simulink model "FSAC2021_V1_Running"  (R2014a)
settings: Solver=FixedStepDiscrete  StartTime=0.0  StopTime=inf  FixedStep=0.0005  RelTol=1e-3
model workspace (MAT data in the model file):
  MCOS : class17 (value not decoded)
  MCOS : class17 (value not decoded)
  MCOS : class17 (value not decoded)
  MCOS : class17 (value not decoded)
  MCOS : class17 (value not decoded)
  MCOS : class17 (value not decoded)
  MCOS : class17 (value not decoded)
  MCOS : class17 (value not decoded)
  MCOS : class17 (value not decoded)
  MCOS : class17 (value not decoded)
  MCOS : class17 (value not decoded)
  MCOS : class17 (value not decoded)
  MCOS : class17 (value not decoded)
  MCOS : class17 (value not decoded)
  MCOS : class17 (value not decoded)
  MCOS : class17 (value not decoded)
  MCOS : class17 (value not decoded)
  MCOS : class17 (value not decoded)
  MCOS : class17 (value not decoded)
  BUZZER_START = 1
  MCOS : class17 (value not decoded)
  MCOS : class17 (value not decoded)
  MCOS : class17 (value not decoded)
  MCOS : class17 (value not decoded)
  MCOS : class17 (value not decoded)
  MCOS : class17 (value not decoded)
  MCOS : class17 (value not decoded)
  MCOS : class17 (value not decoded)
  MCOS : class17 (value not decoded)
  MCOS : class17 (value not decoded)
  MCOS : class17 (value not decoded)
  MCOS : class17 (value not decoded)
  MCOS : class17 (value not decoded)
  MCOS : class17 (value not decoded)
  MCOS : class17 (value not decoded)
  MCOS : class17 (value not decoded)
  MCOS : class17 (value not decoded)
  MCOS : class17 (value not decoded)
  MCOS : class17 (value not decoded)
  MCOS : class17 (value not decoded)
  MCOS : class17 (value not decoded)
  MCOS : class17 (value not decoded)
  MCOS : class17 (value not decoded)
  MCOS : class17 (value not decoded)
  MCOS : class17 (value not decoded)
  MCOS : class17 (value not decoded)
  MCOS : class17 (value not decoded)
  MCOS : class17 (value not decoded)
  MCOS : class17 (value not decoded)
  MCOS : class17 (value not decoded)
  MCOS : class17 (value not decoded)
  MCOS : class17 (value not decoded)
  MCOS : class17 (value not decoded)
  MCOS : class17 (value not decoded)
  MCOS : class17 (value not decoded)
  MCOS : class17 (value not decoded)
  MCOS : class17 (value not decoded)
  MCOS : class17 (value not decoded)
  Brake = 11
  MCOS : class17 (value not decoded)
  MCOS : class17 (value not decoded)
  MCOS : class17 (value not decoded)
  MCOS : class17 (value not decoded)
  MCOS : class17 (value not decoded)
  MCOS : class17 (value not decoded)
  MCOS : class17 (value not decoded)
  MCOS : class17 (value not decoded)
  Sensor_Acc_b = 101.85
  Sensor_Acc_k = -0.0185
  Str_Sen_Orig_Angle = -341
  MCOS : class17 (value not decoded)
  Tire_D = 0.47
  T = 0.05
libraries: simulink x402, ec55xxlib x134
(part 14 of 17)

== system FSAC2021_V1_Running/ROUTING/TO_DCAN/Subsystem/DIAG_BMS_ALARM_RELAY/ALM_DSCH_OCS ==
  ALM_DSCH_OCS : Inport
  ALM_DSCH_OCSRon : Rounding  Operator=round
  ALM_DSCH_OCS_1sat : Saturate  UpperLimit=32  LowerLimit=0
  ALM_DSCH_OCS_Convert : DataTypeConversion  OutDataTypeStr=uint8
  ALM_DSCH_OCS_Convert1 : DataTypeConversion  OutDataTypeStr=uint32
  ALM_DSCH_OCS_D : Product  Inputs=*/
  ALM_DSCH_OCS_F : Constant  OutDataTypeStr=single
  ALM_DSCH_OCS_L : simulink/Logic and Bit Operations/Bitwise Operator  logicop=AND  UseBitMask=on  BitMask=32  BitMaskRealWorld=Stored Integer
  ALM_DSCH_OCS_O : Constant  Value=0  OutDataTypeStr=single
  ALM_DSCH_OCS_S : ArithShift  BitShiftNumber=-5
  ALM_DSCH_OCS_sat : Saturate  UpperLimit=1  LowerLimit=0
  ALM_DSCH_OCS_st : Sum  Inputs=+-
  output2 : Outport
  wires:
  ALM_DSCH_OCS/1 -> ALM_DSCH_OCS_sat/1
  ALM_DSCH_OCS_sat/1 -> ALM_DSCH_OCS_st/1
  ALM_DSCH_OCS_O/1 -> ALM_DSCH_OCS_st/2
  ALM_DSCH_OCS_st/1 -> ALM_DSCH_OCS_D/1
  ALM_DSCH_OCS_F/1 -> ALM_DSCH_OCS_D/2
  ALM_DSCH_OCS_D/1 -> ALM_DSCH_OCSRon/1
  ALM_DSCH_OCSRon/1 -> ALM_DSCH_OCS_S/1
  ALM_DSCH_OCS_S/1 -> ALM_DSCH_OCS_1sat/1
  ALM_DSCH_OCS_1sat/1 -> ALM_DSCH_OCS_Convert1/1
  ALM_DSCH_OCS_Convert1/1 -> ALM_DSCH_OCS_L/1
  ALM_DSCH_OCS_L/1 -> ALM_DSCH_OCS_Convert/1
  ALM_DSCH_OCS_Convert/1 -> output2/1

== system FSAC2021_V1_Running/ROUTING/TO_DCAN/Subsystem/DIAG_BMS_ALARM_RELAY/ALM_DSCH_OCT ==
  ALM_DSCH_OCT : Inport
  ALM_DSCH_OCTRon : Rounding  Operator=round
  ALM_DSCH_OCT_1sat : Saturate  UpperLimit=128  LowerLimit=0
  ALM_DSCH_OCT_Convert : DataTypeConversion  OutDataTypeStr=uint8
  ALM_DSCH_OCT_Convert1 : DataTypeConversion  OutDataTypeStr=uint32
  ALM_DSCH_OCT_D : Product  Inputs=*/
  ALM_DSCH_OCT_F : Constant  OutDataTypeStr=single
  ALM_DSCH_OCT_L : simulink/Logic and Bit Operations/Bitwise Operator  logicop=AND  UseBitMask=on  BitMask=128  BitMaskRealWorld=Stored Integer
  ALM_DSCH_OCT_O : Constant  Value=0  OutDataTypeStr=single
  ALM_DSCH_OCT_S : ArithShift  BitShiftNumber=-7
  ALM_DSCH_OCT_sat : Saturate  UpperLimit=1  LowerLimit=0
  ALM_DSCH_OCT_st : Sum  Inputs=+-
  output2 : Outport
  wires:
  ALM_DSCH_OCT/1 -> ALM_DSCH_OCT_sat/1
  ALM_DSCH_OCT_sat/1 -> ALM_DSCH_OCT_st/1
  ALM_DSCH_OCT_O/1 -> ALM_DSCH_OCT_st/2
  ALM_DSCH_OCT_st/1 -> ALM_DSCH_OCT_D/1
  ALM_DSCH_OCT_F/1 -> ALM_DSCH_OCT_D/2
  ALM_DSCH_OCT_D/1 -> ALM_DSCH_OCTRon/1
  ALM_DSCH_OCTRon/1 -> ALM_DSCH_OCT_S/1
  ALM_DSCH_OCT_S/1 -> ALM_DSCH_OCT_1sat/1
  ALM_DSCH_OCT_1sat/1 -> ALM_DSCH_OCT_Convert1/1
  ALM_DSCH_OCT_Convert1/1 -> ALM_DSCH_OCT_L/1
  ALM_DSCH_OCT_L/1 -> ALM_DSCH_OCT_Convert/1
  ALM_DSCH_OCT_Convert/1 -> output2/1

== system FSAC2021_V1_Running/ROUTING/TO_DCAN/Subsystem/DIAG_BMS_ALARM_RELAY/ALM_HALL_BREAK ==
  ALM_HALL_BREAK : Inport
  ALM_HALL_BREAKRon : Rounding  Operator=round
  ALM_HALL_BREAK_1sat : Saturate  UpperLimit=128  LowerLimit=0
  ALM_HALL_BREAK_Convert : DataTypeConversion  OutDataTypeStr=uint8
  ALM_HALL_BREAK_Convert1 : DataTypeConversion  OutDataTypeStr=uint32
  ALM_HALL_BREAK_D : Product  Inputs=*/
  ALM_HALL_BREAK_F : Constant  OutDataTypeStr=single
  ALM_HALL_BREAK_L : simulink/Logic and Bit Operations/Bitwise Operator  logicop=AND  UseBitMask=on  BitMask=128  BitMaskRealWorld=Stored Integer
  ALM_HALL_BREAK_O : Constant  Value=0  OutDataTypeStr=single
  ALM_HALL_BREAK_S : ArithShift  BitShiftNumber=-7
  ALM_HALL_BREAK_sat : Saturate  UpperLimit=1  LowerLimit=0
  ALM_HALL_BREAK_st : Sum  Inputs=+-
  output3 : Outport
  wires:
  ALM_HALL_BREAK/1 -> ALM_HALL_BREAK_sat/1
  ALM_HALL_BREAK_sat/1 -> ALM_HALL_BREAK_st/1
  ALM_HALL_BREAK_O/1 -> ALM_HALL_BREAK_st/2
  ALM_HALL_BREAK_st/1 -> ALM_HALL_BREAK_D/1
  ALM_HALL_BREAK_F/1 -> ALM_HALL_BREAK_D/2
  ALM_HALL_BREAK_D/1 -> ALM_HALL_BREAKRon/1
  ALM_HALL_BREAKRon/1 -> ALM_HALL_BREAK_S/1
  ALM_HALL_BREAK_S/1 -> ALM_HALL_BREAK_1sat/1
  ALM_HALL_BREAK_1sat/1 -> ALM_HALL_BREAK_Convert1/1
  ALM_HALL_BREAK_Convert1/1 -> ALM_HALL_BREAK_L/1
  ALM_HALL_BREAK_L/1 -> ALM_HALL_BREAK_Convert/1
  ALM_HALL_BREAK_Convert/1 -> output3/1

== system FSAC2021_V1_Running/ROUTING/TO_DCAN/Subsystem/DIAG_BMS_ALARM_RELAY/ALM_HVREL_FAIL ==
  ALM_HVREL_FAIL : Inport
  ALM_HVREL_FAILRon : Rounding  Operator=round
  ALM_HVREL_FAIL_1sat : Saturate  UpperLimit=64  LowerLimit=0
  ALM_HVREL_FAIL_Convert : DataTypeConversion  OutDataTypeStr=uint8
  ALM_HVREL_FAIL_Convert1 : DataTypeConversion  OutDataTypeStr=uint32
  ALM_HVREL_FAIL_D : Product  Inputs=*/
  ALM_HVREL_FAIL_F : Constant  OutDataTypeStr=single
  ALM_HVREL_FAIL_L : simulink/Logic and Bit Operations/Bitwise Operator  logicop=AND  UseBitMask=on  BitMask=64  BitMaskRealWorld=Stored Integer
  ALM_HVREL_FAIL_O : Constant  Value=0  OutDataTypeStr=single
  ALM_HVREL_FAIL_S : ArithShift  BitShiftNumber=-6
  ALM_HVREL_FAIL_sat : Saturate  UpperLimit=1  LowerLimit=0
  ALM_HVREL_FAIL_st : Sum  Inputs=+-
  output3 : Outport
  wires:
  ALM_HVREL_FAIL/1 -> ALM_HVREL_FAIL_sat/1
  ALM_HVREL_FAIL_sat/1 -> ALM_HVREL_FAIL_st/1
  ALM_HVREL_FAIL_O/1 -> ALM_HVREL_FAIL_st/2
  ALM_HVREL_FAIL_st/1 -> ALM_HVREL_FAIL_D/1
  ALM_HVREL_FAIL_F/1 -> ALM_HVREL_FAIL_D/2
  ALM_HVREL_FAIL_D/1 -> ALM_HVREL_FAILRon/1
  ALM_HVREL_FAILRon/1 -> ALM_HVREL_FAIL_S/1
  ALM_HVREL_FAIL_S/1 -> ALM_HVREL_FAIL_1sat/1
  ALM_HVREL_FAIL_1sat/1 -> ALM_HVREL_FAIL_Convert1/1
  ALM_HVREL_FAIL_Convert1/1 -> ALM_HVREL_FAIL_L/1
  ALM_HVREL_FAIL_L/1 -> ALM_HVREL_FAIL_Convert/1
  ALM_HVREL_FAIL_Convert/1 -> output3/1

== system FSAC2021_V1_Running/ROUTING/TO_DCAN/Subsystem/DIAG_BMS_ALARM_RELAY/ALM_LEAK_OC ==
  ALM_LEAK_OC : Inport
  ALM_LEAK_OCRon : Rounding  Operator=round
  ALM_LEAK_OC_1sat : Saturate  UpperLimit=4  LowerLimit=0
  ALM_LEAK_OC_Convert : DataTypeConversion  OutDataTypeStr=uint8
  ALM_LEAK_OC_Convert1 : DataTypeConversion  OutDataTypeStr=uint32
  ALM_LEAK_OC_D : Product  Inputs=*/
  ALM_LEAK_OC_F : Constant  OutDataTypeStr=single
  ALM_LEAK_OC_L : simulink/Logic and Bit Operations/Bitwise Operator  logicop=AND  UseBitMask=on  BitMask=4  BitMaskRealWorld=Stored Integer
  ALM_LEAK_OC_O : Constant  Value=0  OutDataTypeStr=single
  ALM_LEAK_OC_S : ArithShift  BitShiftNumber=-2
  ALM_LEAK_OC_sat : Saturate  UpperLimit=1  LowerLimit=0
  ALM_LEAK_OC_st : Sum  Inputs=+-
  output3 : Outport
  wires:
  ALM_LEAK_OC/1 -> ALM_LEAK_OC_sat/1
  ALM_LEAK_OC_sat/1 -> ALM_LEAK_OC_st/1
  ALM_LEAK_OC_O/1 -> ALM_LEAK_OC_st/2
  ALM_LEAK_OC_st/1 -> ALM_LEAK_OC_D/1
  ALM_LEAK_OC_F/1 -> ALM_LEAK_OC_D/2
  ALM_LEAK_OC_D/1 -> ALM_LEAK_OCRon/1
  ALM_LEAK_OCRon/1 -> ALM_LEAK_OC_S/1
  ALM_LEAK_OC_S/1 -> ALM_LEAK_OC_1sat/1
  ALM_LEAK_OC_1sat/1 -> ALM_LEAK_OC_Convert1/1
  ALM_LEAK_OC_Convert1/1 -> ALM_LEAK_OC_L/1
  ALM_LEAK_OC_L/1 -> ALM_LEAK_OC_Convert/1
  ALM_LEAK_OC_Convert/1 -> output3/1

== system FSAC2021_V1_Running/ROUTING/TO_DCAN/Subsystem/DIAG_BMS_ALARM_RELAY/ALM_PRECHRG_FAIL ==
  ALM_PRECHRG_FAIL : Inport
  ALM_PRECHRG_FAILRon : Rounding  Operator=round
  ALM_PRECHRG_FAIL_1sat : Saturate  UpperLimit=8  LowerLimit=0
  ALM_PRECHRG_FAIL_Convert : DataTypeConversion  OutDataTypeStr=uint8
  ALM_PRECHRG_FAIL_Convert1 : DataTypeConversion  OutDataTypeStr=uint32
  ALM_PRECHRG_FAIL_D : Product  Inputs=*/
  ALM_PRECHRG_FAIL_F : Constant  OutDataTypeStr=single
  ALM_PRECHRG_FAIL_L : simulink/Logic and Bit Operations/Bitwise Operator  logicop=AND  UseBitMask=on  BitMask=8  BitMaskRealWorld=Stored Integer
  ALM_PRECHRG_FAIL_O : Constant  Value=0  OutDataTypeStr=single
  ALM_PRECHRG_FAIL_S : ArithShift  BitShiftNumber=-3
  ALM_PRECHRG_FAIL_sat : Saturate  UpperLimit=1  LowerLimit=0
  ALM_PRECHRG_FAIL_st : Sum  Inputs=+-
  output3 : Outport
  wires:
  ALM_PRECHRG_FAIL/1 -> ALM_PRECHRG_FAIL_sat/1
  ALM_PRECHRG_FAIL_sat/1 -> ALM_PRECHRG_FAIL_st/1
  ALM_PRECHRG_FAIL_O/1 -> ALM_PRECHRG_FAIL_st/2
  ALM_PRECHRG_FAIL_st/1 -> ALM_PRECHRG_FAIL_D/1
  ALM_PRECHRG_FAIL_F/1 -> ALM_PRECHRG_FAIL_D/2
  ALM_PRECHRG_FAIL_D/1 -> ALM_PRECHRG_FAILRon/1
  ALM_PRECHRG_FAILRon/1 -> ALM_PRECHRG_FAIL_S/1
  ALM_PRECHRG_FAIL_S/1 -> ALM_PRECHRG_FAIL_1sat/1
  ALM_PRECHRG_FAIL_1sat/1 -> ALM_PRECHRG_FAIL_Convert1/1
  ALM_PRECHRG_FAIL_Convert1/1 -> ALM_PRECHRG_FAIL_L/1
  ALM_PRECHRG_FAIL_L/1 -> ALM_PRECHRG_FAIL_Convert/1
  ALM_PRECHRG_FAIL_Convert/1 -> output3/1

== system FSAC2021_V1_Running/ROUTING/TO_DCAN/Subsystem/DIAG_BMS_ALARM_RELAY/NegRlyStr ==
  NegRlyStr : Inport
  NegRlyStrRon : Rounding  Operator=round
  NegRlyStr_1sat : Saturate  UpperLimit=12  LowerLimit=0
  NegRlyStr_Convert : DataTypeConversion  OutDataTypeStr=uint8
  NegRlyStr_Convert1 : DataTypeConversion  OutDataTypeStr=uint32
  NegRlyStr_D : Product  Inputs=*/
  NegRlyStr_F : Constant  OutDataTypeStr=single
  NegRlyStr_L : simulink/Logic and Bit Operations/Bitwise Operator  logicop=AND  UseBitMask=on  BitMask=12  BitMaskRealWorld=Stored Integer
  NegRlyStr_O : Constant  Value=0  OutDataTypeStr=single
  NegRlyStr_S : ArithShift  BitShiftNumber=-2
  NegRlyStr_sat : Saturate  UpperLimit=2  LowerLimit=0
  NegRlyStr_st : Sum  Inputs=+-
  output4 : Outport
  wires:
  NegRlyStr/1 -> NegRlyStr_sat/1
  NegRlyStr_sat/1 -> NegRlyStr_st/1
  NegRlyStr_O/1 -> NegRlyStr_st/2
  NegRlyStr_st/1 -> NegRlyStr_D/1
  NegRlyStr_F/1 -> NegRlyStr_D/2
  NegRlyStr_D/1 -> NegRlyStrRon/1
  NegRlyStrRon/1 -> NegRlyStr_S/1
  NegRlyStr_S/1 -> NegRlyStr_1sat/1
  NegRlyStr_1sat/1 -> NegRlyStr_Convert1/1
  NegRlyStr_Convert1/1 -> NegRlyStr_L/1
  NegRlyStr_L/1 -> NegRlyStr_Convert/1
  NegRlyStr_Convert/1 -> output4/1

== system FSAC2021_V1_Running/ROUTING/TO_DCAN/Subsystem/DIAG_BMS_ALARM_RELAY/OnChrRlyStr ==
  OnChrRlyStr : Inport
  OnChrRlyStrRon : Rounding  Operator=round
  OnChrRlyStr_1sat : Saturate  UpperLimit=192  LowerLimit=0
  OnChrRlyStr_Convert : DataTypeConversion  OutDataTypeStr=uint8
  OnChrRlyStr_Convert1 : DataTypeConversion  OutDataTypeStr=uint32
  OnChrRlyStr_D : Product  Inputs=*/
  OnChrRlyStr_F : Constant  OutDataTypeStr=single
  OnChrRlyStr_L : simulink/Logic and Bit Operations/Bitwise Operator  logicop=AND  UseBitMask=on  BitMask=192  BitMaskRealWorld=Stored Integer
  OnChrRlyStr_O : Constant  Value=0  OutDataTypeStr=single
  OnChrRlyStr_S : ArithShift  BitShiftNumber=-6
  OnChrRlyStr_sat : Saturate  UpperLimit=2  LowerLimit=0
  OnChrRlyStr_st : Sum  Inputs=+-
  output4 : Outport
  wires:
  OnChrRlyStr/1 -> OnChrRlyStr_sat/1
  OnChrRlyStr_sat/1 -> OnChrRlyStr_st/1
  OnChrRlyStr_O/1 -> OnChrRlyStr_st/2
  OnChrRlyStr_st/1 -> OnChrRlyStr_D/1
  OnChrRlyStr_F/1 -> OnChrRlyStr_D/2
  OnChrRlyStr_D/1 -> OnChrRlyStrRon/1
  OnChrRlyStrRon/1 -> OnChrRlyStr_S/1
  OnChrRlyStr_S/1 -> OnChrRlyStr_1sat/1
  OnChrRlyStr_1sat/1 -> OnChrRlyStr_Convert1/1
  OnChrRlyStr_Convert1/1 -> OnChrRlyStr_L/1
  OnChrRlyStr_L/1 -> OnChrRlyStr_Convert/1
  OnChrRlyStr_Convert/1 -> output4/1

== system FSAC2021_V1_Running/ROUTING/TO_DCAN/Subsystem/DIAG_BMS_ALARM_RELAY/PosRlyStr ==
  PosRlyStr : Inport
  PosRlyStrRon : Rounding  Operator=round
  PosRlyStr_1sat : Saturate  UpperLimit=3  LowerLimit=0
  PosRlyStr_Convert : DataTypeConversion  OutDataTypeStr=uint8
  PosRlyStr_Convert1 : DataTypeConversion  OutDataTypeStr=uint32
  PosRlyStr_D : Product  Inputs=*/
  PosRlyStr_F : Constant  OutDataTypeStr=single
  PosRlyStr_L : simulink/Logic and Bit Operations/Bitwise Operator  logicop=AND  UseBitMask=on  BitMask=3  BitMaskRealWorld=Stored Integer
  PosRlyStr_O : Constant  Value=0  OutDataTypeStr=single
  PosRlyStr_S : ArithShift
  PosRlyStr_sat : Saturate  UpperLimit=2  LowerLimit=0
  PosRlyStr_st : Sum  Inputs=+-
  output4 : Outport
  wires:
  PosRlyStr/1 -> PosRlyStr_sat/1
  PosRlyStr_sat/1 -> PosRlyStr_st/1
  PosRlyStr_O/1 -> PosRlyStr_st/2
  PosRlyStr_st/1 -> PosRlyStr_D/1
  PosRlyStr_F/1 -> PosRlyStr_D/2
  PosRlyStr_D/1 -> PosRlyStrRon/1
  PosRlyStrRon/1 -> PosRlyStr_S/1
  PosRlyStr_S/1 -> PosRlyStr_1sat/1
  PosRlyStr_1sat/1 -> PosRlyStr_Convert1/1
  PosRlyStr_Convert1/1 -> PosRlyStr_L/1
  PosRlyStr_L/1 -> PosRlyStr_Convert/1
  PosRlyStr_Convert/1 -> output4/1

== system FSAC2021_V1_Running/ROUTING/TO_DCAN/Subsystem/DIAG_BMS_ALARM_RELAY/PreRlyStr ==
  PreRlyStr : Inport
  PreRlyStrRon : Rounding  Operator=round
  PreRlyStr_1sat : Saturate  UpperLimit=48  LowerLimit=0
  PreRlyStr_Convert : DataTypeConversion  OutDataTypeStr=uint8
  PreRlyStr_Convert1 : DataTypeConversion  OutDataTypeStr=uint32
  PreRlyStr_D : Product  Inputs=*/
  PreRlyStr_F : Constant  OutDataTypeStr=single
  PreRlyStr_L : simulink/Logic and Bit Operations/Bitwise Operator  logicop=AND  UseBitMask=on  BitMask=48  BitMaskRealWorld=Stored Integer
  PreRlyStr_O : Constant  Value=0  OutDataTypeStr=single
  PreRlyStr_S : ArithShift  BitShiftNumber=-4
  PreRlyStr_sat : Saturate  UpperLimit=2  LowerLimit=0
  PreRlyStr_st : Sum  Inputs=+-
  output4 : Outport
  wires:
  PreRlyStr/1 -> PreRlyStr_sat/1
  PreRlyStr_sat/1 -> PreRlyStr_st/1
  PreRlyStr_O/1 -> PreRlyStr_st/2
  PreRlyStr_st/1 -> PreRlyStr_D/1
  PreRlyStr_F/1 -> PreRlyStr_D/2
  PreRlyStr_D/1 -> PreRlyStrRon/1
  PreRlyStrRon/1 -> PreRlyStr_S/1
  PreRlyStr_S/1 -> PreRlyStr_1sat/1
  PreRlyStr_1sat/1 -> PreRlyStr_Convert1/1
  PreRlyStr_Convert1/1 -> PreRlyStr_L/1
  PreRlyStr_L/1 -> PreRlyStr_Convert/1
  PreRlyStr_Convert/1 -> output4/1

== system FSAC2021_V1_Running/ROUTING/TO_DCAN/Subsystem/DIAG_BMS_INFO/BatAlmLv ==
  BatAlmLv : Inport
  BatAlmLvRon : Rounding  Operator=round
  BatAlmLv_1sat : Saturate  UpperLimit=15  LowerLimit=0
  BatAlmLv_Convert : DataTypeConversion  OutDataTypeStr=uint8
  BatAlmLv_Convert1 : DataTypeConversion  OutDataTypeStr=uint32
  BatAlmLv_D : Product  Inputs=*/
  BatAlmLv_F : Constant  OutDataTypeStr=single
  BatAlmLv_L : simulink/Logic and Bit Operations/Bitwise Operator  logicop=AND  UseBitMask=on  BitMask=15  BitMaskRealWorld=Stored Integer
  BatAlmLv_O : Constant  Value=0  OutDataTypeStr=single
  BatAlmLv_S : ArithShift
  BatAlmLv_sat : Saturate  UpperLimit=4  LowerLimit=0
  BatAlmLv_st : Sum  Inputs=+-
  output7 : Outport
  wires:
  BatAlmLv/1 -> BatAlmLv_sat/1
  BatAlmLv_sat/1 -> BatAlmLv_st/1
  BatAlmLv_O/1 -> BatAlmLv_st/2
  BatAlmLv_st/1 -> BatAlmLv_D/1
  BatAlmLv_F/1 -> BatAlmLv_D/2
  BatAlmLv_D/1 -> BatAlmLvRon/1
  BatAlmLvRon/1 -> BatAlmLv_S/1
  BatAlmLv_S/1 -> BatAlmLv_1sat/1
  BatAlmLv_1sat/1 -> BatAlmLv_Convert1/1
  BatAlmLv_Convert1/1 -> BatAlmLv_L/1
  BatAlmLv_L/1 -> BatAlmLv_Convert/1
  BatAlmLv_Convert/1 -> output7/1

== system FSAC2021_V1_Running/ROUTING/TO_DCAN/Subsystem/DIAG_BMS_INFO/BatCurrent ==
  BatCurrent : Inport
  BatCurrentBitCov : DataTypeConversion  OutDataTypeStr=uint8
  BatCurrentCOV : DataTypeConversion  OutDataTypeStr=uint8
  BatCurrentRon : Rounding  Operator=round
  BatCurrent_1sat : Saturate  UpperLimit=65535  LowerLimit=0
  BatCurrent_And : simulink/Logic and Bit Operations/Bitwise Operator  logicop=AND  UseBitMask=off  NumInputPorts=2  BitMask=bin2dec('11011001')  BitMaskRealWorld=Stored Integer
  BatCurrent_And_C : Constant  Value=255  OutDataTypeStr=uint32
  BatCurrent_Convert : DataTypeConversion  OutDataTypeStr=uint32
  BatCurrent_D : Product  Inputs=*/
  BatCurrent_D1 : Product  Inputs=*/
  BatCurrent_F : Constant  Value=0.1  OutDataTypeStr=single
  BatCurrent_L : simulink/Logic and Bit Operations/Bitwise Operator  logicop=AND  UseBitMask=on  BitMask=65535  BitMaskRealWorld=Stored Integer
  BatCurrent_O : Constant  Value=-1000  OutDataTypeStr=single
  BatCurrent_S : ArithShift
  BatCurrent_sat : Saturate  UpperLimit=1000  LowerLimit=-1000
  BatCurrent_st : Sum  Inputs=+-
  BatCurrentoutput3_C : Constant  Value=256
  output3 : Outport
  output4 : Outport  Port=2
  wires:
  BatCurrent/1 -> BatCurrent_sat/1
  BatCurrent_sat/1 -> BatCurrent_st/1
  BatCurrent_O/1 -> BatCurrent_st/2
  BatCurrent_st/1 -> BatCurrent_D/1
  BatCurrent_F/1 -> BatCurrent_D/2
  BatCurrent_D/1 -> BatCurrentRon/1
  BatCurrentRon/1 -> BatCurrent_S/1
  BatCurrent_S/1 -> BatCurrent_1sat/1
  BatCurrent_1sat/1 -> BatCurrent_Convert/1
  BatCurrent_Convert/1 -> BatCurrent_L/1
  BatCurrent_L/1 -> BatCurrent_D1/1, BatCurrent_And/1
  BatCurrentoutput3_C/1 -> BatCurrent_D1/2
  BatCurrent_D1/1 -> BatCurrentCOV/1
  BatCurrentCOV/1 -> output3/1
  BatCurrent_And_C/1 -> BatCurrent_And/2
  BatCurrent_And/1 -> BatCurrentBitCov/1
  BatCurrentBitCov/1 -> output4/1

== system FSAC2021_V1_Running/ROUTING/TO_DCAN/Subsystem/DIAG_BMS_INFO/BatLife ==
  BatLife : Inport
  BatLifeRon : Rounding  Operator=round
  BatLife_1sat : Saturate  UpperLimit=255  LowerLimit=0
  BatLife_Convert : DataTypeConversion  OutDataTypeStr=uint8
  BatLife_Convert1 : DataTypeConversion  OutDataTypeStr=uint32
  BatLife_D : Product  Inputs=*/
  BatLife_F : Constant  OutDataTypeStr=single
  BatLife_L : simulink/Logic and Bit Operations/Bitwise Operator  logicop=AND  UseBitMask=on  BitMask=255  BitMaskRealWorld=Stored Integer
  BatLife_O : Constant  Value=0  OutDataTypeStr=single
  BatLife_S : ArithShift
  BatLife_sat : Saturate  UpperLimit=255  LowerLimit=0
  BatLife_st : Sum  Inputs=+-
  output8 : Outport
  wires:
  BatLife/1 -> BatLife_sat/1
  BatLife_sat/1 -> BatLife_st/1
  BatLife_O/1 -> BatLife_st/2
  BatLife_st/1 -> BatLife_D/1
  BatLife_F/1 -> BatLife_D/2
  BatLife_D/1 -> BatLifeRon/1
  BatLifeRon/1 -> BatLife_S/1
  BatLife_S/1 -> BatLife_1sat/1
  BatLife_1sat/1 -> BatLife_Convert1/1
  BatLife_Convert1/1 -> BatLife_L/1
  BatLife_L/1 -> BatLife_Convert/1
  BatLife_Convert/1 -> output8/1

== system FSAC2021_V1_Running/ROUTING/TO_DCAN/Subsystem/DIAG_BMS_INFO/BatSoc ==
  BatSoc : Inport
  BatSocRon : Rounding  Operator=round
  BatSoc_1sat : Saturate  UpperLimit=255  LowerLimit=0
  BatSoc_Convert : DataTypeConversion  OutDataTypeStr=uint8
  BatSoc_Convert1 : DataTypeConversion  OutDataTypeStr=uint32
  BatSoc_D : Product  Inputs=*/
  BatSoc_F : Constant  OutDataTypeStr=single
  BatSoc_L : simulink/Logic and Bit Operations/Bitwise Operator  logicop=AND  UseBitMask=on  BitMask=255  BitMaskRealWorld=Stored Integer
  BatSoc_O : Constant  Value=0  OutDataTypeStr=single
  BatSoc_S : ArithShift
  BatSoc_sat : Saturate  UpperLimit=100  LowerLimit=0
  BatSoc_st : Sum  Inputs=+-
  output5 : Outport
  wires:
  BatSoc/1 -> BatSoc_sat/1
  BatSoc_sat/1 -> BatSoc_st/1
  BatSoc_O/1 -> BatSoc_st/2
  BatSoc_st/1 -> BatSoc_D/1
  BatSoc_F/1 -> BatSoc_D/2
  BatSoc_D/1 -> BatSocRon/1
  BatSocRon/1 -> BatSoc_S/1
  BatSoc_S/1 -> BatSoc_1sat/1
  BatSoc_1sat/1 -> BatSoc_Convert1/1
  BatSoc_Convert1/1 -> BatSoc_L/1
  BatSoc_L/1 -> BatSoc_Convert/1
  BatSoc_Convert/1 -> output5/1

== system FSAC2021_V1_Running/ROUTING/TO_DCAN/Subsystem/DIAG_BMS_INFO/BatSoh ==
  BatSoh : Inport
  BatSohRon : Rounding  Operator=round
  BatSoh_1sat : Saturate  UpperLimit=255  LowerLimit=0
  BatSoh_Convert : DataTypeConversion  OutDataTypeStr=uint8
  BatSoh_Convert1 : DataTypeConversion  OutDataTypeStr=uint32
  BatSoh_D : Product  Inputs=*/
  BatSoh_F : Constant  OutDataTypeStr=single
  BatSoh_L : simulink/Logic and Bit Operations/Bitwise Operator  logicop=AND  UseBitMask=on  BitMask=255  BitMaskRealWorld=Stored Integer
  BatSoh_O : Constant  Value=0  OutDataTypeStr=single
  BatSoh_S : ArithShift
  BatSoh_sat : Saturate  UpperLimit=100  LowerLimit=0
  BatSoh_st : Sum  Inputs=+-
  output6 : Outport
  wires:
  BatSoh/1 -> BatSoh_sat/1
  BatSoh_sat/1 -> BatSoh_st/1
  BatSoh_O/1 -> BatSoh_st/2
  BatSoh_st/1 -> BatSoh_D/1
  BatSoh_F/1 -> BatSoh_D/2
  BatSoh_D/1 -> BatSohRon/1
  BatSohRon/1 -> BatSoh_S/1
  BatSoh_S/1 -> BatSoh_1sat/1
  BatSoh_1sat/1 -> BatSoh_Convert1/1
  BatSoh_Convert1/1 -> BatSoh_L/1
  BatSoh_L/1 -> BatSoh_Convert/1
  BatSoh_Convert/1 -> output6/1

== system FSAC2021_V1_Running/ROUTING/TO_DCAN/Subsystem/DIAG_BMS_INFO/BatState ==
  BatState : Inport
  BatStateRon : Rounding  Operator=round
  BatState_1sat : Saturate  UpperLimit=240  LowerLimit=0
  BatState_Convert : DataTypeConversion  OutDataTypeStr=uint8
  BatState_Convert1 : DataTypeConversion  OutDataTypeStr=uint32
  BatState_D : Product  Inputs=*/
  BatState_F : Constant  OutDataTypeStr=single
  BatState_L : simulink/Logic and Bit Operations/Bitwise Operator  logicop=AND  UseBitMask=on  BitMask=240  BitMaskRealWorld=Stored Integer
  BatState_O : Constant  Value=0  OutDataTypeStr=single
  BatState_S : ArithShift  BitShiftNumber=-4
  BatState_sat : Saturate  UpperLimit=7  LowerLimit=1
  BatState_st : Sum  Inputs=+-
  output7 : Outport
  wires:
  BatState/1 -> BatState_sat/1
  BatState_sat/1 -> BatState_st/1
  BatState_O/1 -> BatState_st/2
  BatState_st/1 -> BatState_D/1
  BatState_F/1 -> BatState_D/2
  BatState_D/1 -> BatStateRon/1
  BatStateRon/1 -> BatState_S/1
  BatState_S/1 -> BatState_1sat/1
  BatState_1sat/1 -> BatState_Convert1/1
  BatState_Convert1/1 -> BatState_L/1
  BatState_L/1 -> BatState_Convert/1
  BatState_Convert/1 -> output7/1

== system FSAC2021_V1_Running/ROUTING/TO_DCAN/Subsystem/DIAG_BMS_INFO/BatVoltage ==
  BatVoltage : Inport
  BatVoltageBitCov : DataTypeConversion  OutDataTypeStr=uint8
  BatVoltageCOV : DataTypeConversion  OutDataTypeStr=uint8
  BatVoltageRon : Rounding  Operator=round
  BatVoltage_1sat : Saturate  UpperLimit=65535  LowerLimit=0
  BatVoltage_And : simulink/Logic and Bit Operations/Bitwise Operator  logicop=AND  UseBitMask=off  NumInputPorts=2  BitMask=bin2dec('11011001')  BitMaskRealWorld=Stored Integer
  BatVoltage_And_C : Constant  Value=255  OutDataTypeStr=uint32
  BatVoltage_Convert : DataTypeConversion  OutDataTypeStr=uint32
  BatVoltage_D : Product  Inputs=*/
  BatVoltage_D1 : Product  Inputs=*/
  BatVoltage_F : Constant  Value=0.1  OutDataTypeStr=single
  BatVoltage_L : simulink/Logic and Bit Operations/Bitwise Operator  logicop=AND  UseBitMask=on  BitMask=65535  BitMaskRealWorld=Stored Integer
  BatVoltage_O : Constant  Value=0  OutDataTypeStr=single
  BatVoltage_S : ArithShift
  BatVoltage_sat : Saturate  UpperLimit=900  LowerLimit=0
  BatVoltage_st : Sum  Inputs=+-
  BatVoltageoutput1_C : Constant  Value=256
  output1 : Outport
  output2 : Outport  Port=2
  wires:
  BatVoltage/1 -> BatVoltage_sat/1
  BatVoltage_sat/1 -> BatVoltage_st/1
  BatVoltage_O/1 -> BatVoltage_st/2
  BatVoltage_st/1 -> BatVoltage_D/1
  BatVoltage_F/1 -> BatVoltage_D/2
  BatVoltage_D/1 -> BatVoltageRon/1
  BatVoltageRon/1 -> BatVoltage_S/1
  BatVoltage_S/1 -> BatVoltage_1sat/1
  BatVoltage_1sat/1 -> BatVoltage_Convert/1
  BatVoltage_Convert/1 -> BatVoltage_L/1
  BatVoltage_L/1 -> BatVoltage_D1/1, BatVoltage_And/1
  BatVoltageoutput1_C/1 -> BatVoltage_D1/2
  BatVoltage_D1/1 -> BatVoltageCOV/1
  BatVoltageCOV/1 -> output1/1
  BatVoltage_And_C/1 -> BatVoltage_And/2
  BatVoltage_And/1 -> BatVoltageBitCov/1
  BatVoltageBitCov/1 -> output2/1

== system FSAC2021_V1_Running/ROUTING/TO_DCAN/Subsystem/DIAG_BMS_MAXT/MaxTemp ==
  MaxTemp : Inport
  MaxTempRon : Rounding  Operator=round
  MaxTemp_1sat : Saturate  UpperLimit=255  LowerLimit=0
  MaxTemp_Convert : DataTypeConversion  OutDataTypeStr=uint8
  MaxTemp_Convert1 : DataTypeConversion  OutDataTypeStr=uint32
  MaxTemp_D : Product  Inputs=*/
  MaxTemp_F : Constant  OutDataTypeStr=single
  MaxTemp_L : simulink/Logic and Bit Operations/Bitwise Operator  logicop=AND  UseBitMask=on  BitMask=255  BitMaskRealWorld=Stored Integer
  MaxTemp_O : Constant  Value=-40  OutDataTypeStr=single
  MaxTemp_S : ArithShift
  MaxTemp_sat : Saturate  UpperLimit=120  LowerLimit=-40
  MaxTemp_st : Sum  Inputs=+-
  output1 : Outport
  wires:
  MaxTemp/1 -> MaxTemp_sat/1
  MaxTemp_sat/1 -> MaxTemp_st/1
  MaxTemp_O/1 -> MaxTemp_st/2
  MaxTemp_st/1 -> MaxTemp_D/1
  MaxTemp_F/1 -> MaxTemp_D/2
  MaxTemp_D/1 -> MaxTempRon/1
  MaxTempRon/1 -> MaxTemp_S/1
  MaxTemp_S/1 -> MaxTemp_1sat/1
  MaxTemp_1sat/1 -> MaxTemp_Convert1/1
  MaxTemp_Convert1/1 -> MaxTemp_L/1
  MaxTemp_L/1 -> MaxTemp_Convert/1
  MaxTemp_Convert/1 -> output1/1

== system FSAC2021_V1_Running/ROUTING/TO_DCAN/Subsystem/DIAG_BMS_MAXT/MaxTempNo ==
  MaxTempNo : Inport
  MaxTempNoRon : Rounding  Operator=round
  MaxTempNo_1sat : Saturate  UpperLimit=255  LowerLimit=0
  MaxTempNo_Convert : DataTypeConversion  OutDataTypeStr=uint8
  MaxTempNo_Convert1 : DataTypeConversion  OutDataTypeStr=uint32
  MaxTempNo_D : Product  Inputs=*/
  MaxTempNo_F : Constant  OutDataTypeStr=single
  MaxTempNo_L : simulink/Logic and Bit Operations/Bitwise Operator  logicop=AND  UseBitMask=on  BitMask=255  BitMaskRealWorld=Stored Integer
  MaxTempNo_O : Constant  Value=0  OutDataTypeStr=single
  MaxTempNo_S : ArithShift
  MaxTempNo_sat : Saturate  UpperLimit=255  LowerLimit=0
  MaxTempNo_st : Sum  Inputs=+-
  output3 : Outport
  wires:
  MaxTempNo/1 -> MaxTempNo_sat/1
  MaxTempNo_sat/1 -> MaxTempNo_st/1
  MaxTempNo_O/1 -> MaxTempNo_st/2
  MaxTempNo_st/1 -> MaxTempNo_D/1
  MaxTempNo_F/1 -> MaxTempNo_D/2
  MaxTempNo_D/1 -> MaxTempNoRon/1
  MaxTempNoRon/1 -> MaxTempNo_S/1
  MaxTempNo_S/1 -> MaxTempNo_1sat/1
  MaxTempNo_1sat/1 -> MaxTempNo_Convert1/1
  MaxTempNo_Convert1/1 -> MaxTempNo_L/1
  MaxTempNo_L/1 -> MaxTempNo_Convert/1
  MaxTempNo_Convert/1 -> output3/1

== system FSAC2021_V1_Running/ROUTING/TO_DCAN/Subsystem/DIAG_BMS_MAXT/MinTemp ==
  MinTemp : Inport
  MinTempRon : Rounding  Operator=round
  MinTemp_1sat : Saturate  UpperLimit=255  LowerLimit=0
  MinTemp_Convert : DataTypeConversion  OutDataTypeStr=uint8
  MinTemp_Convert1 : DataTypeConversion  OutDataTypeStr=uint32
  MinTemp_D : Product  Inputs=*/
  MinTemp_F : Constant  OutDataTypeStr=single
  MinTemp_L : simulink/Logic and Bit Operations/Bitwise Operator  logicop=AND  UseBitMask=on  BitMask=255  BitMaskRealWorld=Stored Integer
  MinTemp_O : Constant  Value=-40  OutDataTypeStr=single
  MinTemp_S : ArithShift
  MinTemp_sat : Saturate  UpperLimit=120  LowerLimit=-40
  MinTemp_st : Sum  Inputs=+-
  output2 : Outport
  wires:
  MinTemp/1 -> MinTemp_sat/1
  MinTemp_sat/1 -> MinTemp_st/1
  MinTemp_O/1 -> MinTemp_st/2
  MinTemp_st/1 -> MinTemp_D/1
  MinTemp_F/1 -> MinTemp_D/2
  MinTemp_D/1 -> MinTempRon/1
  MinTempRon/1 -> MinTemp_S/1
  MinTemp_S/1 -> MinTemp_1sat/1
  MinTemp_1sat/1 -> MinTemp_Convert1/1
  MinTemp_Convert1/1 -> MinTemp_L/1
  MinTemp_L/1 -> MinTemp_Convert/1
  MinTemp_Convert/1 -> output2/1

== system FSAC2021_V1_Running/ROUTING/TO_DCAN/Subsystem/DIAG_BMS_MAXT/MinTempNo ==
  MinTempNo : Inport
  MinTempNoRon : Rounding  Operator=round
  MinTempNo_1sat : Saturate  UpperLimit=255  LowerLimit=0
  MinTempNo_Convert : DataTypeConversion  OutDataTypeStr=uint8
  MinTempNo_Convert1 : DataTypeConversion  OutDataTypeStr=uint32
  MinTempNo_D : Product  Inputs=*/
  MinTempNo_F : Constant  OutDataTypeStr=single
  MinTempNo_L : simulink/Logic and Bit Operations/Bitwise Operator  logicop=AND  UseBitMask=on  BitMask=255  BitMaskRealWorld=Stored Integer
  MinTempNo_O : Constant  Value=0  OutDataTypeStr=single
  MinTempNo_S : ArithShift
  MinTempNo_sat : Saturate  UpperLimit=255  LowerLimit=0
  MinTempNo_st : Sum  Inputs=+-
  output4 : Outport
  wires:
  MinTempNo/1 -> MinTempNo_sat/1
  MinTempNo_sat/1 -> MinTempNo_st/1
  MinTempNo_O/1 -> MinTempNo_st/2
  MinTempNo_st/1 -> MinTempNo_D/1
  MinTempNo_F/1 -> MinTempNo_D/2
  MinTempNo_D/1 -> MinTempNoRon/1
  MinTempNoRon/1 -> MinTempNo_S/1
  MinTempNo_S/1 -> MinTempNo_1sat/1
  MinTempNo_1sat/1 -> MinTempNo_Convert1/1
  MinTempNo_Convert1/1 -> MinTempNo_L/1
  MinTempNo_L/1 -> MinTempNo_Convert/1
  MinTempNo_Convert/1 -> output4/1

== system FSAC2021_V1_Running/ROUTING/TO_DCAN/Subsystem/DIAG_BMS_MAXV/MaxCellVolt ==
  MaxCellVolt : Inport
  MaxCellVoltBitCov : DataTypeConversion  OutDataTypeStr=uint8
  MaxCellVoltCOV : DataTypeConversion  OutDataTypeStr=uint8
  MaxCellVoltRon : Rounding  Operator=round
  MaxCellVolt_1sat : Saturate  UpperLimit=65535  LowerLimit=0
  MaxCellVolt_And : simulink/Logic and Bit Operations/Bitwise Operator  logicop=AND  UseBitMask=off  NumInputPorts=2  BitMask=bin2dec('11011001')  BitMaskRealWorld=Stored Integer
  MaxCellVolt_And_C : Constant  Value=255  OutDataTypeStr=uint32
  MaxCellVolt_Convert : DataTypeConversion  OutDataTypeStr=uint32
  MaxCellVolt_D : Product  Inputs=*/
  MaxCellVolt_D1 : Product  Inputs=*/
  MaxCellVolt_F : Constant  OutDataTypeStr=single
  MaxCellVolt_L : simulink/Logic and Bit Operations/Bitwise Operator  logicop=AND  UseBitMask=on  BitMask=65535  BitMaskRealWorld=Stored Integer
  MaxCellVolt_O : Constant  Value=0  OutDataTypeStr=single
  MaxCellVolt_S : ArithShift
  MaxCellVolt_sat : Saturate  UpperLimit=5000  LowerLimit=0
  MaxCellVolt_st : Sum  Inputs=+-
  MaxCellVoltoutput1_C : Constant  Value=256
  output1 : Outport
  output2 : Outport  Port=2
  wires:
  MaxCellVolt/1 -> MaxCellVolt_sat/1
  MaxCellVolt_sat/1 -> MaxCellVolt_st/1
  MaxCellVolt_O/1 -> MaxCellVolt_st/2
  MaxCellVolt_st/1 -> MaxCellVolt_D/1
  MaxCellVolt_F/1 -> MaxCellVolt_D/2
  MaxCellVolt_D/1 -> MaxCellVoltRon/1
  MaxCellVoltRon/1 -> MaxCellVolt_S/1
  MaxCellVolt_S/1 -> MaxCellVolt_1sat/1
  MaxCellVolt_1sat/1 -> MaxCellVolt_Convert/1
  MaxCellVolt_Convert/1 -> MaxCellVolt_L/1
  MaxCellVolt_L/1 -> MaxCellVolt_D1/1, MaxCellVolt_And/1
  MaxCellVoltoutput1_C/1 -> MaxCellVolt_D1/2
  MaxCellVolt_D1/1 -> MaxCellVoltCOV/1
  MaxCellVoltCOV/1 -> output1/1
  MaxCellVolt_And_C/1 -> MaxCellVolt_And/2
  MaxCellVolt_And/1 -> MaxCellVoltBitCov/1
  MaxCellVoltBitCov/1 -> output2/1

== system FSAC2021_V1_Running/ROUTING/TO_DCAN/Subsystem/DIAG_BMS_MAXV/MaxCellVoltNo ==
  MaxCellVoltNo : Inport
  MaxCellVoltNoRon : Rounding  Operator=round
  MaxCellVoltNo_1sat : Saturate  UpperLimit=255  LowerLimit=0
  MaxCellVoltNo_Convert : DataTypeConversion  OutDataTypeStr=uint8
  MaxCellVoltNo_Convert1 : DataTypeConversion  OutDataTypeStr=uint32
  MaxCellVoltNo_D : Product  Inputs=*/
  MaxCellVoltNo_F : Constant  OutDataTypeStr=single
  MaxCellVoltNo_L : simulink/Logic and Bit Operations/Bitwise Operator  logicop=AND  UseBitMask=on  BitMask=255  BitMaskRealWorld=Stored Integer
  MaxCellVoltNo_O : Constant  Value=0  OutDataTypeStr=single
  MaxCellVoltNo_S : ArithShift
  MaxCellVoltNo_sat : Saturate  UpperLimit=255  LowerLimit=0
  MaxCellVoltNo_st : Sum  Inputs=+-
  output6 : Outport
  wires:
  MaxCellVoltNo/1 -> MaxCellVoltNo_sat/1
  MaxCellVoltNo_sat/1 -> MaxCellVoltNo_st/1
  MaxCellVoltNo_O/1 -> MaxCellVoltNo_st/2
  MaxCellVoltNo_st/1 -> MaxCellVoltNo_D/1
  MaxCellVoltNo_F/1 -> MaxCellVoltNo_D/2
  MaxCellVoltNo_D/1 -> MaxCellVoltNoRon/1
  MaxCellVoltNoRon/1 -> MaxCellVoltNo_S/1
  MaxCellVoltNo_S/1 -> MaxCellVoltNo_1sat/1
  MaxCellVoltNo_1sat/1 -> MaxCellVoltNo_Convert1/1
  MaxCellVoltNo_Convert1/1 -> MaxCellVoltNo_L/1
  MaxCellVoltNo_L/1 -> MaxCellVoltNo_Convert/1
  MaxCellVoltNo_Convert/1 -> output6/1

== system FSAC2021_V1_Running/ROUTING/TO_DCAN/Subsystem/DIAG_BMS_MAXV/MinCellVolt ==
  MinCellVolt : Inport
  MinCellVoltBitCov : DataTypeConversion  OutDataTypeStr=uint8
  MinCellVoltCOV : DataTypeConversion  OutDataTypeStr=uint8
  MinCellVoltRon : Rounding  Operator=round
  MinCellVolt_1sat : Saturate  UpperLimit=65535  LowerLimit=0
  MinCellVolt_And : simulink/Logic and Bit Operations/Bitwise Operator  logicop=AND  UseBitMask=off  NumInputPorts=2  BitMask=bin2dec('11011001')  BitMaskRealWorld=Stored Integer
  MinCellVolt_And_C : Constant  Value=255  OutDataTypeStr=uint32
  MinCellVolt_Convert : DataTypeConversion  OutDataTypeStr=uint32
  MinCellVolt_D : Product  Inputs=*/
  MinCellVolt_D1 : Product  Inputs=*/
  MinCellVolt_F : Constant  OutDataTypeStr=single
  MinCellVolt_L : simulink/Logic and Bit Operations/Bitwise Operator  logicop=AND  UseBitMask=on  BitMask=65535  BitMaskRealWorld=Stored Integer
  MinCellVolt_O : Constant  Value=0  OutDataTypeStr=single
  MinCellVolt_S : ArithShift
  MinCellVolt_sat : Saturate  UpperLimit=5000  LowerLimit=0
  MinCellVolt_st : Sum  Inputs=+-
  MinCellVoltoutput3_C : Constant  Value=256
  output3 : Outport
  output4 : Outport  Port=2
  wires:
  MinCellVolt/1 -> MinCellVolt_sat/1
  MinCellVolt_sat/1 -> MinCellVolt_st/1
  MinCellVolt_O/1 -> MinCellVolt_st/2
  MinCellVolt_st/1 -> MinCellVolt_D/1
  MinCellVolt_F/1 -> MinCellVolt_D/2
  MinCellVolt_D/1 -> MinCellVoltRon/1
  MinCellVoltRon/1 -> MinCellVolt_S/1
  MinCellVolt_S/1 -> MinCellVolt_1sat/1
  MinCellVolt_1sat/1 -> MinCellVolt_Convert/1
  MinCellVolt_Convert/1 -> MinCellVolt_L/1
  MinCellVolt_L/1 -> MinCellVolt_D1/1, MinCellVolt_And/1
  MinCellVoltoutput3_C/1 -> MinCellVolt_D1/2
  MinCellVolt_D1/1 -> MinCellVoltCOV/1
  MinCellVoltCOV/1 -> output3/1
  MinCellVolt_And_C/1 -> MinCellVolt_And/2
  MinCellVolt_And/1 -> MinCellVoltBitCov/1
  MinCellVoltBitCov/1 -> output4/1

== system FSAC2021_V1_Running/ROUTING/TO_DCAN/Subsystem/DIAG_BMS_MAXV/MinCellVoltNo ==
  MinCellVoltNo : Inport
  MinCellVoltNoRon : Rounding  Operator=round
  MinCellVoltNo_1sat : Saturate  UpperLimit=255  LowerLimit=0
  MinCellVoltNo_Convert : DataTypeConversion  OutDataTypeStr=uint8
  MinCellVoltNo_Convert1 : DataTypeConversion  OutDataTypeStr=uint32
  MinCellVoltNo_D : Product  Inputs=*/
  MinCellVoltNo_F : Constant  OutDataTypeStr=single
  MinCellVoltNo_L : simulink/Logic and Bit Operations/Bitwise Operator  logicop=AND  UseBitMask=on  BitMask=255  BitMaskRealWorld=Stored Integer
  MinCellVoltNo_O : Constant  Value=0  OutDataTypeStr=single
  MinCellVoltNo_S : ArithShift
  MinCellVoltNo_sat : Saturate  UpperLimit=255  LowerLimit=0
  MinCellVoltNo_st : Sum  Inputs=+-
  output5 : Outport
  wires:
  MinCellVoltNo/1 -> MinCellVoltNo_sat/1
  MinCellVoltNo_sat/1 -> MinCellVoltNo_st/1
  MinCellVoltNo_O/1 -> MinCellVoltNo_st/2
  MinCellVoltNo_st/1 -> MinCellVoltNo_D/1
  MinCellVoltNo_F/1 -> MinCellVoltNo_D/2
  MinCellVoltNo_D/1 -> MinCellVoltNoRon/1
  MinCellVoltNoRon/1 -> MinCellVoltNo_S/1
  MinCellVoltNo_S/1 -> MinCellVoltNo_1sat/1
  MinCellVoltNo_1sat/1 -> MinCellVoltNo_Convert1/1
  MinCellVoltNo_Convert1/1 -> MinCellVoltNo_L/1
  MinCellVoltNo_L/1 -> MinCellVoltNo_Convert/1
  MinCellVoltNo_Convert/1 -> output5/1

== system FSAC2021_V1_Running/ROUTING/TO_DCAN/Subsystem/DIAG_RES_INFO/RES_ACC ==
  RES_ACC : Inport
  Constant{1..2,4..8} (7 alike) : Constant  Value=0  OutDataTypeStr=uint8  SampleTime=-1
  RES_ACCRon : Rounding  Operator=round
  RES_ACC_1sat : Saturate  UpperLimit=255  LowerLimit=0
  RES_ACC_Convert : DataTypeConversion  OutDataTypeStr=uint8
  RES_ACC_Convert1 : DataTypeConversion  OutDataTypeStr=uint32
  RES_ACC_D : Product  Inputs=*/
  RES_ACC_F : Constant  OutDataTypeStr=single
  RES_ACC_L : simulink/Logic and Bit Operations/Bitwise Operator  logicop=AND  UseBitMask=on  BitMask=255  BitMaskRealWorld=Stored Integer
  RES_ACC_O : Constant  Value=0  OutDataTypeStr=single
  RES_ACC_S : ArithShift
  RES_ACC_sat : Saturate  UpperLimit=100  LowerLimit=0
  RES_ACC_st : Sum  Inputs=+-
  output1 : Outport
  output2 : Outport  Port=2
  output3 : Outport  Port=3
  output4 : Outport  Port=4
  output5 : Outport  Port=5
  output6 : Outport  Port=6
  output7 : Outport  Port=7
  output8 : Outport  Port=8
  wires:
  RES_ACC/1 -> RES_ACC_sat/1
  RES_ACC_sat/1 -> RES_ACC_st/1
  RES_ACC_O/1 -> RES_ACC_st/2
  RES_ACC_st/1 -> RES_ACC_D/1
  RES_ACC_F/1 -> RES_ACC_D/2
  RES_ACC_D/1 -> RES_ACCRon/1
  RES_ACCRon/1 -> RES_ACC_S/1
  RES_ACC_S/1 -> RES_ACC_1sat/1
  RES_ACC_1sat/1 -> RES_ACC_Convert1/1
  RES_ACC_Convert1/1 -> RES_ACC_L/1
  RES_ACC_L/1 -> RES_ACC_Convert/1
  RES_ACC_Convert/1 -> output3/1
  Constant1/1 -> output1/1
  Constant2/1 -> output2/1
  Constant4/1 -> output4/1
  Constant5/1 -> output5/1
  Constant6/1 -> output6/1
  Constant7/1 -> output7/1
  Constant8/1 -> output8/1

== system FSAC2021_V1_Running/ROUTING/TO_DCAN/Subsystem/DIAG_RES_INFO/RES_Brake ==
  RES_Brake : Inport
  Constant{1,3..8} (7 alike) : Constant  Value=0  OutDataTypeStr=uint8  SampleTime=-1
  RES_BrakeRon : Rounding  Operator=round
  RES_Brake_1sat : Saturate  UpperLimit=255  LowerLimit=0
  RES_Brake_Convert : DataTypeConversion  OutDataTypeStr=uint8
  RES_Brake_Convert1 : DataTypeConversion  OutDataTypeStr=uint32
  RES_Brake_D : Product  Inputs=*/
  RES_Brake_F : Constant  OutDataTypeStr=single
  RES_Brake_L : simulink/Logic and Bit Operations/Bitwise Operator  logicop=AND  UseBitMask=on  BitMask=255  BitMaskRealWorld=Stored Integer
  RES_Brake_O : Constant  Value=0  OutDataTypeStr=single
  RES_Brake_S : ArithShift
  RES_Brake_sat : Saturate  UpperLimit=100  LowerLimit=0
  RES_Brake_st : Sum  Inputs=+-
  output1 : Outport
  output2 : Outport  Port=2
  output3 : Outport  Port=3
  output4 : Outport  Port=4
  output5 : Outport  Port=5
  output6 : Outport  Port=6
  output7 : Outport  Port=7
  output8 : Outport  Port=8
  wires:
  RES_Brake/1 -> RES_Brake_sat/1
  RES_Brake_sat/1 -> RES_Brake_st/1
  RES_Brake_O/1 -> RES_Brake_st/2
  RES_Brake_st/1 -> RES_Brake_D/1
  RES_Brake_F/1 -> RES_Brake_D/2
  RES_Brake_D/1 -> RES_BrakeRon/1
  RES_BrakeRon/1 -> RES_Brake_S/1
  RES_Brake_S/1 -> RES_Brake_1sat/1
  RES_Brake_1sat/1 -> RES_Brake_Convert1/1
  RES_Brake_Convert1/1 -> RES_Brake_L/1
  RES_Brake_L/1 -> RES_Brake_Convert/1
  RES_Brake_Convert/1 -> output2/1
  Constant1/1 -> output1/1
  Constant3/1 -> output3/1
  Constant4/1 -> output4/1
  Constant5/1 -> output5/1
  Constant6/1 -> output6/1
  Constant7/1 -> output7/1
  Constant8/1 -> output8/1

== system FSAC2021_V1_Running/ROUTING/TO_DCAN/Subsystem/DIAG_RES_INFO/RES_EBS ==
  RES_EBS : Inport
  Constant{1..3,5..8} (7 alike) : Constant  Value=0  OutDataTypeStr=uint8  SampleTime=-1
  RES_EBSRon : Rounding  Operator=round
  RES_EBS_1sat : Saturate  UpperLimit=4  LowerLimit=0
  RES_EBS_Convert : DataTypeConversion  OutDataTypeStr=uint8
  RES_EBS_Convert1 : DataTypeConversion  OutDataTypeStr=uint32
  RES_EBS_D : Product  Inputs=*/
  RES_EBS_F : Constant  OutDataTypeStr=single
  RES_EBS_L : simulink/Logic and Bit Operations/Bitwise Operator  logicop=AND  UseBitMask=on  BitMask=4  BitMaskRealWorld=Stored Integer
  RES_EBS_O : Constant  Value=0  OutDataTypeStr=single
  RES_EBS_S : ArithShift  BitShiftNumber=-2
  RES_EBS_sat : Saturate  UpperLimit=1  LowerLimit=0
  RES_EBS_st : Sum  Inputs=+-
  output1 : Outport
  output2 : Outport  Port=2
  output3 : Outport  Port=3
  output4 : Outport  Port=4
  output5 : Outport  Port=5
  output6 : Outport  Port=6
  output7 : Outport  Port=7
  output8 : Outport  Port=8
  wires:
  RES_EBS/1 -> RES_EBS_sat/1
  RES_EBS_sat/1 -> RES_EBS_st/1
  RES_EBS_O/1 -> RES_EBS_st/2
  RES_EBS_st/1 -> RES_EBS_D/1
  RES_EBS_F/1 -> RES_EBS_D/2
  RES_EBS_D/1 -> RES_EBSRon/1
  RES_EBSRon/1 -> RES_EBS_S/1
  RES_EBS_S/1 -> RES_EBS_1sat/1
  RES_EBS_1sat/1 -> RES_EBS_Convert1/1
  RES_EBS_Convert1/1 -> RES_EBS_L/1
  RES_EBS_L/1 -> RES_EBS_Convert/1
  RES_EBS_Convert/1 -> output4/1
  Constant1/1 -> output1/1
  Constant2/1 -> output2/1
  Constant3/1 -> output3/1
  Constant5/1 -> output5/1
  Constant6/1 -> output6/1
  Constant7/1 -> output7/1
  Constant8/1 -> output8/1

== system FSAC2021_V1_Running/ROUTING/TO_DCAN/Subsystem/DIAG_RES_INFO/RES_GO ==
  RES_GO : Inport
  Constant{1..3,5..8} (7 alike) : Constant  Value=0  OutDataTypeStr=uint8  SampleTime=-1
  RES_GORon : Rounding  Operator=round
  RES_GO_1sat : Saturate  UpperLimit=2  LowerLimit=0
  RES_GO_Convert : DataTypeConversion  OutDataTypeStr=uint8
  RES_GO_Convert1 : DataTypeConversion  OutDataTypeStr=uint32
  RES_GO_D : Product  Inputs=*/
  RES_GO_F : Constant  OutDataTypeStr=single
  RES_GO_L : simulink/Logic and Bit Operations/Bitwise Operator  logicop=AND  UseBitMask=on  BitMask=2  BitMaskRealWorld=Stored Integer
  RES_GO_O : Constant  Value=0  OutDataTypeStr=single
  RES_GO_S : ArithShift  BitShiftNumber=-1
  RES_GO_sat : Saturate  UpperLimit=1  LowerLimit=0
  RES_GO_st : Sum  Inputs=+-
  output1 : Outport
  output2 : Outport  Port=2
  output3 : Outport  Port=3
  output4 : Outport  Port=4
  output5 : Outport  Port=5
  output6 : Outport  Port=6
  output7 : Outport  Port=7
  output8 : Outport  Port=8
  wires:
  RES_GO/1 -> RES_GO_sat/1
  RES_GO_sat/1 -> RES_GO_st/1
  RES_GO_O/1 -> RES_GO_st/2
  RES_GO_st/1 -> RES_GO_D/1
  RES_GO_F/1 -> RES_GO_D/2
  RES_GO_D/1 -> RES_GORon/1
  RES_GORon/1 -> RES_GO_S/1
  RES_GO_S/1 -> RES_GO_1sat/1
  RES_GO_1sat/1 -> RES_GO_Convert1/1
  RES_GO_Convert1/1 -> RES_GO_L/1
  RES_GO_L/1 -> RES_GO_Convert/1
  RES_GO_Convert/1 -> output4/1
  Constant1/1 -> output1/1
  Constant2/1 -> output2/1
  Constant3/1 -> output3/1
  Constant5/1 -> output5/1
  Constant6/1 -> output6/1
  Constant7/1 -> output7/1
  Constant8/1 -> output8/1

== system FSAC2021_V1_Running/ROUTING/TO_DCAN/Subsystem/DIAG_RES_INFO/RES_Return_INFO ==
  RES_Return_INFO : Inport
  Constant{1..3,5..8} (7 alike) : Constant  Value=0  OutDataTypeStr=uint8  SampleTime=-1
  RES_Return_INFORon : Rounding  Operator=round
  RES_Return_INFO_1sat : Saturate  UpperLimit=1  LowerLimit=0
  RES_Return_INFO_Convert : DataTypeConversion  OutDataTypeStr=uint8
  RES_Return_INFO_Convert1 : DataTypeConversion  OutDataTypeStr=uint32
  RES_Return_INFO_D : Product  Inputs=*/
  RES_Return_INFO_F : Constant  OutDataTypeStr=single
  RES_Return_INFO_L : simulink/Logic and Bit Operations/Bitwise Operator  logicop=AND  UseBitMask=on  BitMask=1  BitMaskRealWorld=Stored Integer
  RES_Return_INFO_O : Constant  Value=0  OutDataTypeStr=single
  RES_Return_INFO_S : ArithShift
  RES_Return_INFO_sat : Saturate  UpperLimit=0  LowerLimit=0
  RES_Return_INFO_st : Sum  Inputs=+-
  output1 : Outport
  output2 : Outport  Port=2
  output3 : Outport  Port=3
  output4 : Outport  Port=4
  output5 : Outport  Port=5
  output6 : Outport  Port=6
  output7 : Outport  Port=7
  output8 : Outport  Port=8
  wires:
  RES_Return_INFO/1 -> RES_Return_INFO_sat/1
  RES_Return_INFO_sat/1 -> RES_Return_INFO_st/1
  RES_Return_INFO_O/1 -> RES_Return_INFO_st/2
  RES_Return_INFO_st/1 -> RES_Return_INFO_D/1
  RES_Return_INFO_F/1 -> RES_Return_INFO_D/2
  RES_Return_INFO_D/1 -> RES_Return_INFORon/1
  RES_Return_INFORon/1 -> RES_Return_INFO_S/1
  RES_Return_INFO_S/1 -> RES_Return_INFO_1sat/1
  RES_Return_INFO_1sat/1 -> RES_Return_INFO_Convert1/1
  RES_Return_INFO_Convert1/1 -> RES_Return_INFO_L/1
  RES_Return_INFO_L/1 -> RES_Return_INFO_Convert/1
  RES_Return_INFO_Convert/1 -> output4/1
  Constant1/1 -> output1/1
  Constant2/1 -> output2/1
  Constant3/1 -> output3/1
  Constant5/1 -> output5/1
  Constant6/1 -> output6/1
  Constant7/1 -> output7/1
  Constant8/1 -> output8/1

== system FSAC2021_V1_Running/ROUTING/TO_DCAN/Subsystem/DIAG_RES_INFO/RES_Steering ==
  RES_Steering : Inport
  Constant{2..8} (7 alike) : Constant  Value=0  OutDataTypeStr=uint8  SampleTime=-1
  RES_SteeringABS : Abs
  RES_SteeringCS : ArithShift  BitShiftNumber=-8
  RES_SteeringConS : Constant  OutDataTypeStr=single
  RES_SteeringCosR : Constant  Value=0  OutDataTypeStr=uint8
  RES_SteeringROP : RelationalOperator  Operator=<  OutDataTypeStr=boolean
  RES_SteeringRon : Rounding  Operator=round
  RES_SteeringSW : Switch  Criteria=u2 ~= 0
  RES_Steering_1sat : Saturate  UpperLimit=255  LowerLimit=0
  RES_Steering_Convert : DataTypeConversion  OutDataTypeStr=uint8
  RES_Steering_Convert1 : DataTypeConversion  OutDataTypeStr=uint32
  RES_Steering_D : Product  Inputs=*/
  RES_Steering_F : Constant  OutDataTypeStr=single
  RES_Steering_L : simulink/Logic and Bit Operations/Bitwise Operator  logicop=AND  UseBitMask=on  BitMask=255  BitMaskRealWorld=Stored Integer
  RES_Steering_O : Constant  Value=0  OutDataTypeStr=single
  RES_Steering_S : ArithShift
  RES_Steering_sat : Saturate  UpperLimit=120  LowerLimit=-120
  RES_Steering_st : Sum  Inputs=+-
  RES_Steeringsubcon : Sum  Inputs=+-
  output1 : Outport
  output2 : Outport  Port=2
  output3 : Outport  Port=3
  output4 : Outport  Port=4
  output5 : Outport  Port=5
  output6 : Outport  Port=6
  output7 : Outport  Port=7
  output8 : Outport  Port=8
  wires:
  RES_Steering/1 -> RES_Steering_sat/1
  RES_Steering_sat/1 -> RES_Steering_st/1
  RES_Steering_O/1 -> RES_Steering_st/2
  RES_Steering_st/1 -> RES_Steering_D/1
  RES_Steering_F/1 -> RES_Steering_D/2
  RES_Steering_D/1 -> RES_SteeringRon/1
  RES_SteeringRon/1 -> RES_SteeringROP/1, RES_SteeringABS/1, RES_SteeringSW/3
  RES_SteeringCosR/1 -> RES_SteeringROP/2
  RES_SteeringConS/1 -> RES_SteeringCS/1
  RES_SteeringCS/1 -> RES_Steeringsubcon/1
  RES_SteeringABS/1 -> RES_Steeringsubcon/2
  RES_Steeringsubcon/1 -> RES_SteeringSW/1
  RES_SteeringROP/1 -> RES_SteeringSW/2
  RES_SteeringSW/1 -> RES_Steering_S/1
  RES_Steering_S/1 -> RES_Steering_1sat/1
  RES_Steering_1sat/1 -> RES_Steering_Convert1/1
  RES_Steering_Convert1/1 -> RES_Steering_L/1
  RES_Steering_L/1 -> RES_Steering_Convert/1
  RES_Steering_Convert/1 -> output1/1
  Constant2/1 -> output2/1
  Constant3/1 -> output3/1
  Constant4/1 -> output4/1
  Constant5/1 -> output5/1
  Constant6/1 -> output6/1
  Constant7/1 -> output7/1
  Constant8/1 -> output8/1

== system FSAC2021_V1_Running/ROUTING/TO_DCAN/Subsystem/DIAG_SCU/Fault ==
  Fault : Inport
  FaultRon : Rounding  Operator=round
  Fault_1sat : Saturate  UpperLimit=32  LowerLimit=0
  Fault_Convert : DataTypeConversion  OutDataTypeStr=uint8
  Fault_Convert1 : DataTypeConversion  OutDataTypeStr=uint32
  Fault_D : Product  Inputs=*/
  Fault_F : Constant  OutDataTypeStr=single
  Fault_L : simulink/Logic and Bit Operations/Bitwise Operator  logicop=AND  UseBitMask=on  BitMask=32  BitMaskRealWorld=Stored Integer
  Fault_O : Constant  Value=0  OutDataTypeStr=single
  Fault_S : ArithShift  BitShiftNumber=-5
  Fault_sat : Saturate  UpperLimit=0  LowerLimit=0
  Fault_st : Sum  Inputs=+-
  output5 : Outport
  wires:
  Fault/1 -> Fault_sat/1
  Fault_sat/1 -> Fault_st/1
  Fault_O/1 -> Fault_st/2
  Fault_st/1 -> Fault_D/1
  Fault_F/1 -> Fault_D/2
  Fault_D/1 -> FaultRon/1
  FaultRon/1 -> Fault_S/1
  Fault_S/1 -> Fault_1sat/1
  Fault_1sat/1 -> Fault_Convert1/1
  Fault_Convert1/1 -> Fault_L/1
  Fault_L/1 -> Fault_Convert/1
  Fault_Convert/1 -> output5/1
